simulink model "SimNL"  (R2016b)
settings: Solver=VariableStepAuto  StartTime=0.0  StopTime=10  FixedStep=SampleTime  RelTol=1e-3
libraries: AircraftModel x1
settings Model: Creator=Paul Freeman  LastModifiedBy=rega0051
settings DataIOCC: SignalLoggingSaveFormat=ModelDataLogs  SaveState=on
settings OptimizationCC: ExpressionDepthLimit=2147483647  LifeSpan=inf
settings DebuggingCC: AlgebraicLoopMsg=none  SaveWithParameterizedLinksMsg=none  UnderspecifiedInitializationDetection=Classic  MergeDetectMultiDrivingBlocksExec=none  FcnCallInpInsideContextMsg=warning  UnconnectedInputMsg=none  UnconnectedOutputMsg=none  UnconnectedLineMsg=none  StateNameClashWarn=warning  SFUnexpectedBacktrackingDiag=warning  SFNoUnconditionalDefaultTransitionDiag=warning  SFExecutionAtInitializationDiag=none
settings HardwareCC: ProdBitPerPointer=32  ProdBitPerSizeT=32  ProdBitPerPtrDiffT=32  ProdLargestAtomicFloat=None  ProdIntDivRoundTo=Undefined  ProdEndianess=Unspecified  ProdWordSize=32  ProdHWDeviceType=32-bit Generic
settings ModelReferenceCC: PropagateSignalLabelsOutOfModel=off
settings GRTTargetCC: TargetLangStandard=C89/C90 (ANSI)  GeneratePreprocessorConditionals=Disable all  CombineOutputUpdateFcns=off  GRTInterface=on
settings ConfigComp: CovMetricSettings=dw  CovHtmlReporting=on  CovSaveCumulativeToWorkspaceVar=on  CovSaveSingleToWorkspaceVar=on  CovExternalEMLEnable=off  CovSFcnEnable=off

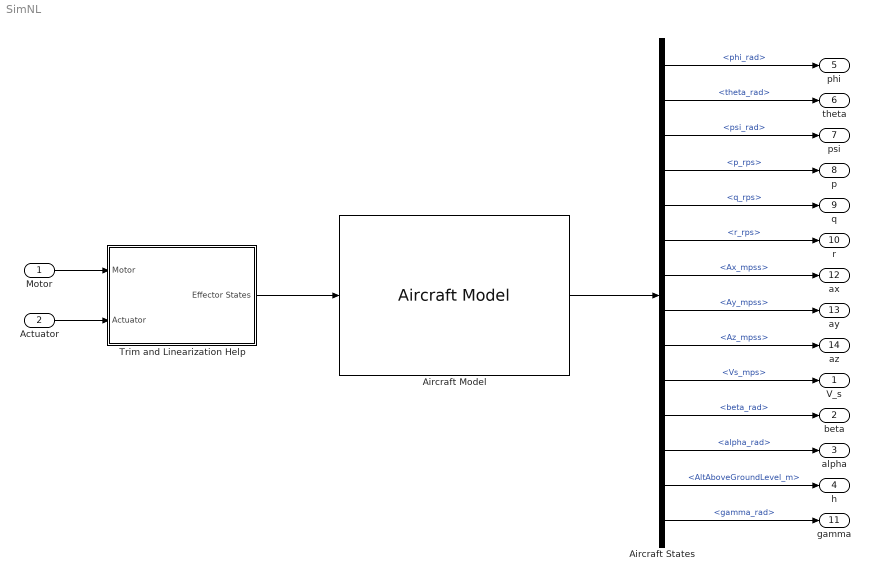
== system SimNL ==
  Motor : Inport
  Actuator : Inport  Port=2
  Aircraft Model : AircraftModel/Aircraft Model
  Aircraft States : BusSelector  OutputSignals=RigidStates.Euler.phi_rad,RigidStates.Euler.theta_rad,RigidStates.Euler.psi_rad,RigidStates.AngVel.p_rps,RigidStates.AngVel.q_rps,RigidStates.AngVel.r_rps,RigidStates.Accels.Ax_mpss,RigidStates.Accels.Ay_mpss,RigidStates.Accels.Az_mpss,AuxVar.WindAxesParams.Vs_mps,AuxVar.WindAxesParams.beta_rad,AuxVar.WindAxesParams.alpha_rad,AuxVar.Nav.AltAboveGroundLevel_m,AuxVar.Nav.gamma_rad
  Trim and Linearization Help : Subsystem
  V_s : Outport
  beta : Outport  Port=2
  alpha : Outport  Port=3
  h : Outport  Port=4
  phi : Outport  Port=5
  theta : Outport  Port=6
  psi : Outport  Port=7
  p : Outport  Port=8
  q : Outport  Port=9
  r : Outport  Port=10
  gamma : Outport  Port=11
  ax : Outport  Port=12
  ay : Outport  Port=13
  az : Outport  Port=14
  wires:
  Aircraft Model/1 -> Aircraft States/1
  Aircraft States/1 -> phi/1  "<phi_rad>"
  Aircraft States/2 -> theta/1  "<theta_rad>"
  Aircraft States/3 -> psi/1  "<psi_rad>"
  Aircraft States/4 -> p/1  "<p_rps>"
  Aircraft States/5 -> q/1  "<q_rps>"
  Aircraft States/6 -> r/1  "<r_rps>"
  Aircraft States/7 -> ax/1  "<Ax_mpss>"
  Aircraft States/8 -> ay/1  "<Ay_mpss>"
  Aircraft States/9 -> az/1  "<Az_mpss>"
  Aircraft States/10 -> V_s/1  "<Vs_mps>"
  Aircraft States/12 -> alpha/1  "<alpha_rad>"
  Aircraft States/14 -> gamma/1  "<gamma_rad>"
  Aircraft States/13 -> h/1  "<AltAboveGroundLevel_m>"
  Aircraft States/11 -> beta/1  "<beta_rad>"
  Actuator/1 -> Trim and Linearization Help/2(Actuator)
  Trim and Linearization Help/1(Effector States) -> Aircraft Model/1
  Motor/1 -> Trim and Linearization Help/1(Motor)

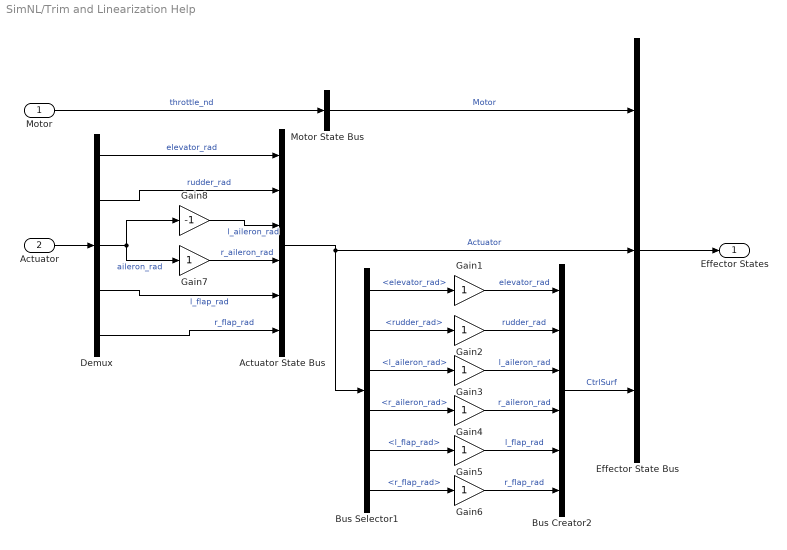
== system SimNL/Trim and Linearization Help ==
  Motor : Inport
  Actuator : Inport  Port=2
  Actuator State Bus : BusCreator  Inputs=6  OutDataTypeStr=Bus: Actuator
  Bus Creator2 : BusCreator  Inputs=6  OutDataTypeStr=Bus: CtrlSurf
      settings: InheritFromInputs=off
  Bus Selector1 : BusSelector  OutputSignals=elevator_rad,rudder_rad,l_aileron_rad,r_aileron_rad,l_flap_rad,r_flap_rad
  Demux : Demux  Outputs=5
  Effector State Bus : BusCreator  Inputs=3  OutDataTypeStr=Bus: Effectors
      settings: InheritFromInputs=off
  Gain{1..7} (7 alike) : Gain
  Gain8 : Gain  Gain=-1
  Motor State Bus : BusCreator  Inputs=1  OutDataTypeStr=Bus: Motor
  Effector States : Outport  OutDataTypeStr=Bus: Effectors
  wires:
  Motor/1 -> Motor State Bus/1  "throttle_nd"
  Demux/2 -> Actuator State Bus/2  "rudder_rad"
  Demux/1 -> Actuator State Bus/1  "elevator_rad"
  Actuator/1 -> Demux/1
  Demux/5 -> Actuator State Bus/6  "r_flap_rad"
  Demux/3 -> Gain8/1, Gain7/1  "aileron_rad"
  Effector State Bus/1 -> Effector States/1
  Actuator State Bus/1 -> Effector State Bus/2, Bus Selector1/1  "Actuator"
  Bus Selector1/1 -> Gain1/1  "<elevator_rad>"
  Bus Selector1/2 -> Gain2/1  "<rudder_rad>"
  Bus Selector1/3 -> Gain3/1  "<l_aileron_rad>"
  Bus Selector1/6 -> Gain6/1  "<r_flap_rad>"
  Gain1/1 -> Bus Creator2/1  "elevator_rad"
  Gain2/1 -> Bus Creator2/2  "rudder_rad"
  Gain3/1 -> Bus Creator2/3  "l_aileron_rad"
  Gain4/1 -> Bus Creator2/4  "r_aileron_rad"
  Gain5/1 -> Bus Creator2/5  "l_flap_rad"
  Gain6/1 -> Bus Creator2/6  "r_flap_rad"
  Bus Creator2/1 -> Effector State Bus/3  "CtrlSurf"
  Demux/4 -> Actuator State Bus/5  "l_flap_rad"
  Gain7/1 -> Actuator State Bus/4  "r_aileron_rad"
  Gain8/1 -> Actuator State Bus/3  "l_aileron_rad"
  Bus Selector1/5 -> Gain5/1  "<l_flap_rad>"
  Bus Selector1/4 -> Gain4/1  "<r_aileron_rad>"
  Motor State Bus/1 -> Effector State Bus/1  "Motor"
